simulink model "fromWorkSpace_TestGen15"  (R2017b)
settings: Solver=FixedStepDiscrete  StartTime=0.0  StopTime=10.0  RelTol=1e-3
model workspace (MAT data in the model file):
  X_structure.time = [0; 0.2; 0.4; 0.6; 0.8; 1; 1.2; 1.4; 1.6; 1.8; 2; 2.2; 2.4; 2.6; 2.8; 3; 3.2; 3.4; 3.6; 3.8; 4; 4.2; 4.4; 4.6; 4.8; 5; 5.2; 5.4; 5.6; 5.8; 6; 6.2; 6.4; 6.6; 6.8; 7; 7.2; 7.4; 7.6; 7.8; 8; 8.2; 8.4; 8.6; 8.8; 9; 9.2; 9.4; 9.6; 9.8]
  X_structure.signals.values = [0 0.198669330795 0.389418342309 0.564642473395 0.7173560909 0.841470984808 0.932039085967 0.985449729988 0.999573603042 0.973847630878 0.909297426826 0.80849640382 ... (150 elements, 50x3)]
  X_structure.signals.dimensions = 3
settings Model: Creator=ktrinh  LastModifiedBy=ktrinh
settings DebuggingCC: ParameterOverflowMsg=none

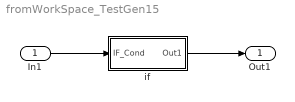
== system fromWorkSpace_TestGen15 ==
  In1 : Inport
  if : Subsystem  AncestorBlock=Block_TestLib/if
  Out1 : Outport
  wires:
  In1/1 -> if/1(IF_Cond)
  if/1(Out1) -> Out1/1

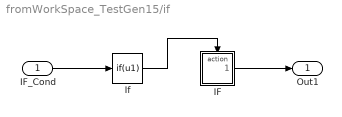
== system fromWorkSpace_TestGen15/if ==
  IF_Cond : Inport  OutDataTypeStr=boolean
  IF : Subsystem  TreatAsAtomicUnit=on
  If : If  IfExpression=u1  ShowElse=off
  Out1 : Outport
  wires:
  If/1 -> IF/Action
  IF_Cond/1 -> If/1
  IF/1(Out1) -> Out1/1

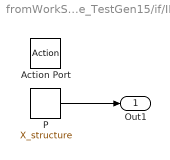
== system fromWorkSpace_TestGen15/if/IF ==
  Action Port : ActionPort  ActionType=then
  P : FromWorkspace  VariableName=X_structure  Interpolate=off  OutputAfterFinalValue=Holding final value
  Out1 : Outport
  wires:
  P/1 -> Out1/1
